simulink model "Step_5"  (Simulink 7.2)
settings: Solver=ode23t  StartTime=0.0  StopTime=inf  FixedStep=0.1  MaxStep=1  RelTol=1e-3
model workspace (MAT data in the model file):
  k = 0.01
  h0 = 1
  r2h : num (value not decoded)
PreLoadFcn:
  | bdclose all
libraries: simulink x5, sfWorkshop_libs x2, gaugeslibv2 x1
settings Model: Creator=wcampbel  LastModifiedBy=wcampbel
settings OptimizationCC: InitFltsAndDblsToZero=on

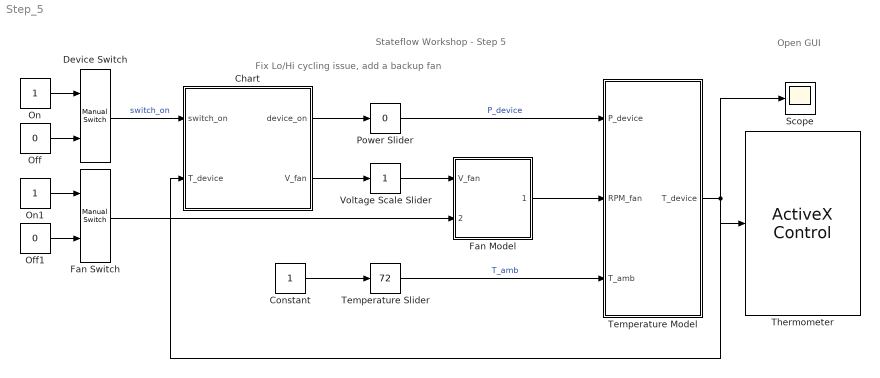
== system Step_5 ==
  note: Stateflow Workshop - Step 5
  note: Fix Lo/Hi cycling issue, add a backup fan
  note: Open GUI
  Chart : Stateflow chart
  Constant : Constant  OutDataType=sfix(16)  OutScaling=2^0
  Device Switch : simulink/Signal Routing/Manual Switch  SystemSampleTime=-1  sw=0  action=0  varsize=off
  Fan Model : Subsystem  BlockChoice=Advanced
      settings: TemplateBlock=sfWorkshop_libs/Fan Model  MemberBlocks=Advanced,Simple
  Fan Switch : simulink/Signal Routing/Manual Switch  SystemSampleTime=-1  sw=1  action=0  varsize=off
  Off : Constant  Value=0  OutDataType=sfix(16)  OutScaling=2^0
  Off1 : Constant  Value=0  OutDataType=sfix(16)  OutScaling=2^0
  On : Constant  OutDataType=sfix(16)  OutScaling=2^0
  On1 : Constant  OutDataType=sfix(16)  OutScaling=2^0
  Power Slider : simulink/Math Operations/Slider Gain  SystemSampleTime=-1  low=0  gain=0  high=400
  Scope : Scope
  Temperature Model : Subsystem  BlockChoice=(Pace Control)
      settings: TemplateBlock=sfWorkshop_libs/Temperature Model  MemberBlocks=(No Pace Control),(Pace Control)
  Temperature Slider : simulink/Math Operations/Slider Gain  SystemSampleTime=-1  low=0  gain=72  high=125
  Thermometer : gaugeslibv2/ActiveX Control  Tag=000  progid=mwslider.sliderctrl.1  connect=input  input=Value  init=hActx.configuration='Slider\Thermometer'; hActx.MouseControl = 'NoMouseControl';  inblock=on  border=on  updateParam=0
  Voltage Scale Slider : simulink/Math Operations/Slider Gain  SystemSampleTime=-1  low=0  gain=1  high=2
  wires:
  On/1 -> Device Switch/1
  Off/1 -> Device Switch/2
  Constant/1 -> Temperature Slider/1
  Device Switch/1 -> Chart/1(switch_on)  "switch_on"
  Chart/2(V_fan) -> Voltage Scale Slider/1
  Temperature Model/1(T_device) -> Scope/1, Chart/2(T_device), Thermometer/1
  Power Slider/1 -> Temperature Model/1(P_device)  "P_device"
  Temperature Slider/1 -> Temperature Model/3(T_amb)  "T_amb"
  Fan Model/1(RPM_fan) -> Temperature Model/2(RPM_fan)
  Voltage Scale Slider/1 -> Fan Model/1(V_fan)
  On1/1 -> Fan Switch/1
  Off1/1 -> Fan Switch/2
  Fan Switch/1 -> Fan Model/2(Override)
  Chart/1(device_on) -> Power Slider/1

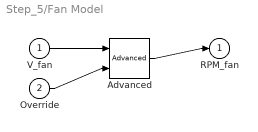
== system Step_5/Fan Model ==
  V_fan : Inport
  Override : Inport  Port=2
  Advanced : sfWorkshop_libs/Advanced  SystemSampleTime=-1
  RPM_fan : Outport
  wires:
  V_fan/1 -> Advanced/1
  Override/1 -> Advanced/2
  Advanced/1 -> RPM_fan/1

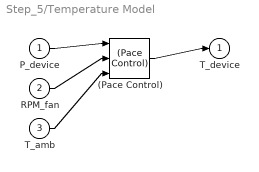
== system Step_5/Temperature Model ==
  P_device : Inport
  RPM_fan : Inport  Port=2
  T_amb : Inport  Port=3
  (Pace Control) : sfWorkshop_libs/(Pace Control)  SystemSampleTime=-1
  T_device : Outport
  wires:
  P_device/1 -> (Pace Control)/1
  RPM_fan/1 -> (Pace Control)/2
  T_amb/1 -> (Pace Control)/3
  (Pace Control)/1 -> T_device/1

== stateflow chart Chart ==
  state DeviceLogic [parallel]
    settings: executionOrder=1
    state DeviceOn
      entry: device_on = 1;
      during: FanTable(T_device)
    state DeviceOff
      entry: device_on = 0;
    DeviceOff -> DeviceOn : [switch_on && isCool(T_device)]
    DeviceOn -> DeviceOff : [!switch_on || !isCool(T_device)]
        | {fan_mode = 0;}
    (default) -> DeviceOff
  state FanTable(T) [function]
    (default) -> (junction 14)
    (junction 14) -> (junction 15) : {
        | /* Device is cold */
        | aVarTruthTableCondition_1 = (T < 50);
        | }
    (junction 15) -> (junction 16) : {
        | /* Device is lukewarm */
        | aVarTruthTableCondition_2 = (T < 120);
        | }
    (junction 16) -> (junction 17) : {
        | /* Device is warm */
        | aVarTruthTableCondition_3 = (T < 160);
        | }
    (junction 17) -> (junction 18) [order 1] : [aVarTruthTableCondition_1]
    (junction 18) -> (junction 19) : {
        | /* 'A1':no fan (too cold or too hot) */
        | fan_mode = 0;
        | }
    (junction 17) -> (junction 20) [order 2]
    (junction 20) -> (junction 21) [order 1] : [aVarTruthTableCondition_2]
    (junction 21) -> (junction 22) : {
        | /* 'A2':low fan */
        | fan_mode = 1;
        | }
    (junction 20) -> (junction 23) [order 2]
    (junction 23) -> (junction 24) [order 1] : [aVarTruthTableCondition_3]
    (junction 24) -> (junction 25) : {
        | /* 'A3':high fan */
        | fan_mode = 2;
        | }
    (junction 23) -> (junction 26) [order 2]
    (junction 26) -> (junction 27) : /* Default */
    (junction 27) -> (junction 28) : {
        | /* 'A1':no fan (too cold or too hot) */
        | fan_mode = 0;
        | }
  state FanLogic [parallel]
    settings: executionOrder=2
    state FanOff
      entry: V_fan[idx] = 0;
    state FanLo
      entry: V_fan[idx] = 0.75;
    state FanHi
      entry: V_fan[idx] = 1.0;
    (default) -> FanOff : {idx = 0;}
    FanOff -> FanLo [order 1] : [fan_mode == 1]
    FanLo -> FanOff [order 2] : [fan_mode == 0 && after(60,sec)]
    FanHi -> FanLo [order 1] : [fan_mode == 1 && after(60,sec)]
    FanLo -> FanHi [order 1] : [fan_mode == 2]
    FanHi -> FanOff [order 2] : [fan_mode == 0]
    FanOff -> FanHi [order 2] : [fan_mode == 2]
  state status = isCool(T) [function]
    (junction 13) -> (junction 12) [order 2] : {status = 0;}
    (junction 13) -> (junction 12) [order 1] : [T<=160]{status = 1;}
    (default) -> (junction 13)
  data: T function_input double; aVarTruthTableCondition_1 temporary boolean =0; aVarTruthTableCondition_2 temporary boolean =0; aVarTruthTableCondition_3 temporary boolean =0; status function_output double; T function_input double; device_on output double; switch_on input double; T_device input double; V_fan output double size=2; fan_mode local double; idx local double
  data aVarTruthTableCondition_1 settings: description=Device is cold
  data aVarTruthTableCondition_2 settings: description=Device is lukewarm
  data aVarTruthTableCondition_3 settings: description=Device is warm
